simulink model "te10_07_es23_simulink"  (R2025b)
settings: Solver=VariableStepAuto  StartTime=0.0  StopTime=10  RelTol=1e-3
settings Model: Creator=robert  LastModifiedBy=robert

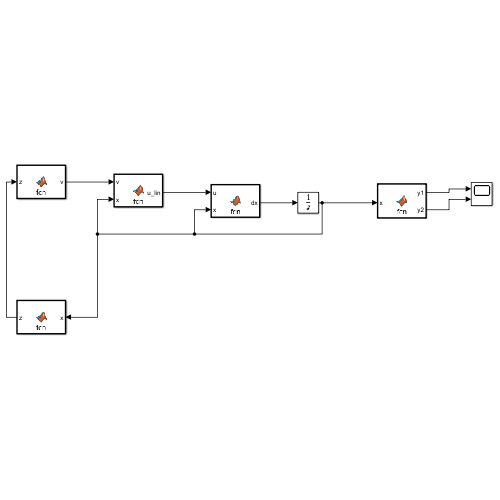
[thumbnail: Simulink's stored preview of the top-level diagram]
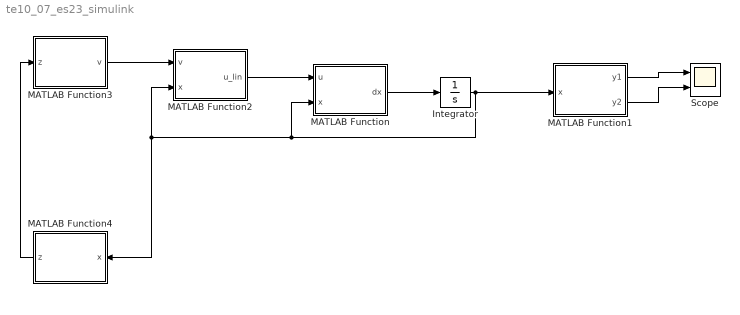
== system te10_07_es23_simulink ==
  Integrator : Integrator  InitialCondition=[3; 5]
  MATLAB Function : MATLAB Function  TreatAsAtomicUnit=on
  MATLAB Function1 : MATLAB Function  TreatAsAtomicUnit=on
  MATLAB Function2 : MATLAB Function  TreatAsAtomicUnit=on
  MATLAB Function3 : MATLAB Function  TreatAsAtomicUnit=on
  MATLAB Function4 : MATLAB Function  TreatAsAtomicUnit=on
  Scope : Scope  NumInputPorts=2
      settings: ActiveDisplayYMinimum=-3.1247318381597973  ActiveDisplayYMaximum=28.124970204239979
  wires:
  MATLAB Function/1(dx) -> Integrator/1
  Integrator/1 -> MATLAB Function4/1(x), MATLAB Function2/2(x), MATLAB Function/2(x), MATLAB Function1/1(x)
  MATLAB Function1/1(y1) -> Scope/1
  MATLAB Function2/1(u_lin) -> MATLAB Function/1(u)
  MATLAB Function3/1(v) -> MATLAB Function2/1(v)
  MATLAB Function4/1(z) -> MATLAB Function3/1(z)
  MATLAB Function1/2(y2) -> Scope/2

== matlab function te10_07_es23_simulink/MATLAB Function ==
  data: u input; dx output; x input
function dx = fcn(u, x)

x1 = x(1);
x2 = x(2);

dx = [3*(x1^2 + x1)*x2; -4*x2 + x1 - x2*u + 3*u];

== matlab function te10_07_es23_simulink/MATLAB Function2 ==
  data: v input; u_lin output; x input
function u_lin = fcn(v,x)
x1 = x(1);
x2 = x(2);

u_lin = ((6*x1^2 + 6*x1)*(x1 - 4*x2) - v + 2*x2^2*(6*x1 + 3)*(3*x1^2 + 3*x1))/((6*x1^2 + 6*x1)*(x2 - 3));

== matlab function te10_07_es23_simulink/MATLAB Function3 ==
  data: z input; v output
function v = fcn(z)
z1 = z(1);
z2 = z(2);

K = [12.5000 7.5000];
v = -K(1)*z(2) - K(2)*z(2);

== matlab function te10_07_es23_simulink/MATLAB Function4 ==
  data: x input; z output
function z = fcn(x)
x1 = x(1);
x2 = x(2);
z = [2*x1;2*x2*(3*x1^2 + 3*x1)];

== matlab function te10_07_es23_simulink/MATLAB Function1 ==
  data: y1 output; x input; y2 output
function [y1,y2] = fcn(x)

y1 = 5*x(2);
y2 = 2*x(1);
